simulink model "ssc_sselecpowersrc"  (R2015a)
settings: Solver=ode15s  StartTime=0.0  StopTime=3600  RelTol=1e-3
InitFcn:
  | if ~exist('E_NOM_KWH', 'var')
  |     E_NOM_KWH = 20;
  |     V_NOM = 400;
  |     E_INIT_KWH = 0.1*E_NOM_KWH;
  | end
  | 
  | C = E_NOM_KWH*3.6e6/V_NOM^2;
  | V0 = V_NOM * sqrt(2*E_INIT_KWH/E_NOM_KWH)
StopFcn:
  | clear C V0
libraries: fl_lib x7, nesl_utility x5, sselecpowersrclib x1
settings Model: Creator=e102261  LastModifiedBy=e102261
settings DataIOCC: SaveOutput=off  SignalLogging=off  DSMLogging=off  VisualizeSimOutput=off  SaveTime=off

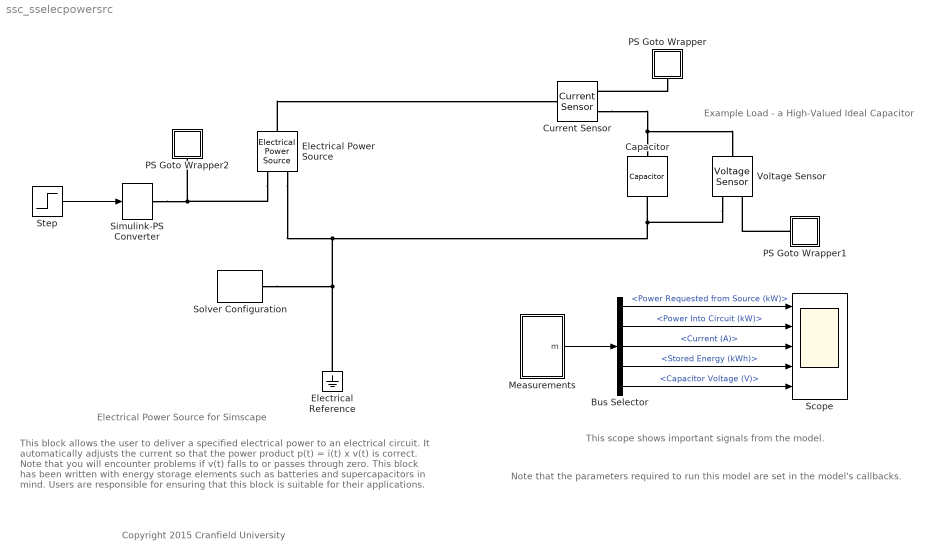
== system ssc_sselecpowersrc ==
  note: Note that the parameters required to run this model are set in the model's callbacks.
  note: This scope shows important signals from the model.
  note: Example Load - a High-Valued Ideal Capacitor
  note: This block allows the user to deliver a specified electrical power to an electrical
      | circuit. It automatically adjusts the current so that the power product
      | p(t) = i(t) x v(t) is correct.  Note that you will encounter problems if v(t) falls to or
      | passes through zero. This block has been written with energy storage elements
      | such as batteries and supercapacitors in mind. Users are responsible for
      | ensuring that this block is suitable for their applications.
  note: Copyright 2015 Cranfield University
  note: Electrical Power Source for Simscape
  Bus Selector : BusSelector  OutputSignals=Power Requested from Source (kW),Power Into Circuit (kW),Current (A),Stored Energy (kWh),Capacitor Voltage (V)
  Capacitor : fl_lib/Electrical/Electrical Elements/Capacitor  c=C F  r=0 Ohm  g=0 1/Ohm  i_specify=off  i_priority=High  i=0 A  v_specify=on  v_priority=High  v=V0 V  vc_specify=off  vc_priority=High  vc=0 V
  Current Sensor : fl_lib/Electrical/Electrical Sensors/Current Sensor
  Electrical Power Source : sselecpowersrclib/Electrical Power Source
  Electrical Reference : fl_lib/Electrical/Electrical Elements/Electrical Reference
  Measurements : Subsystem
  PS Goto Wrapper : Subsystem
  PS Goto Wrapper1 : Subsystem
  PS Goto Wrapper2 : Subsystem
  Scope : Scope  NumInputPorts=5
      settings: TimeRange=3600  YMin=0~0~0~0~0  YMax=20~20~100~10~400
  Simulink-PS Converter : nesl_utility/Simulink-PS Converter  PhysicalDomain=network_engine_domain  SubClassName=ps_input  LeftPortType=input  RightPortType=output  PseudoPeriodic=off  Frequencies=[]  NoiseDistribution=none  NoiseParameters=[]  Unit=W  AffineConversion=off  InputFiltering=off  SimscapeFilterOrder=1  InputFilterTimeConstant=0.001  UdotUserProvided=1
  Solver Configuration : nesl_utility/Solver Configuration  PhysicalDomain=network_engine_domain  SubClassName=solver  LeftPortType=input  RightPortType=generic  Accelerate=off  Tones=[]  Harmonics=[]  SimulateNoise=off  Profile=off  UseLocalSampling=off  EnableSwitchedLinearOptims=on  FrequencyDomain=off  UseCCode=off  RelTol=0.001  AbsTol=1e-06  MinStep=1e-09  ToWorkspace=off  RevertToSquareIcSolve=off  NumHomotopyIterations=100  DoDC=off  ResidualTolerance=1e-09  UseLocalSolver=off  LocalSolverChoice=NE_BACKWARD_EULER_ADVANCER  LocalSolverSampleTime=0.001  DoFixedCost=off  MaxNonlinIter=3  MaxModeIter=2  LinearAlgebra=Sparse  DelaysMemoryBudget=1024  AutomaticFiltering=on  FilteringTimeConstant=0.001
  Step : Step  Time=720  After=E_NOM_KWH/2*1e3  SampleTime=0
  Voltage Sensor : fl_lib/Electrical/Electrical Sensors/Voltage Sensor
  wires:
  Step/1 -> Simulink-PS Converter/1
  Measurements/1(m) -> Bus Selector/1
  Bus Selector/2 -> Scope/2  "<Power Into Circuit (kW)>"
  Bus Selector/1 -> Scope/1  "<Power Requested from Source (kW)>"
  Bus Selector/4 -> Scope/4  "<Stored Energy (kWh)>"
  Bus Selector/3 -> Scope/3  "<Current (A)>"
  Bus Selector/5 -> Scope/5  "<Capacitor Voltage (V)>"
  connections:
  Voltage Sensor/RConn2 -- Electrical Power Source/LConn2 -- Electrical Reference/LConn1 -- Solver Configuration/RConn1 -- Capacitor/RConn1
  Current Sensor/RConn2 -- Voltage Sensor/LConn1 -- Capacitor/LConn1
  PS Goto Wrapper1/LConn1 -- Voltage Sensor/RConn1
  Electrical Power Source/RConn1 -- Current Sensor/LConn1
  Simulink-PS Converter/RConn1 -- Electrical Power Source/LConn1 -- PS Goto Wrapper2/LConn1
  PS Goto Wrapper/LConn1 -- Current Sensor/RConn1

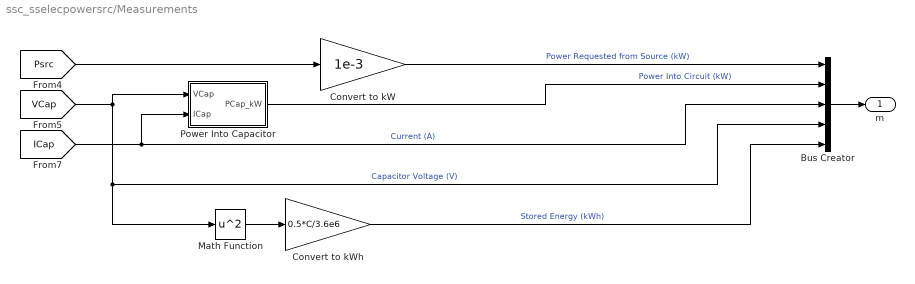
== system ssc_sselecpowersrc/Measurements ==
  Bus Creator : BusCreator  Inputs=5
  Convert to kW : Gain  Gain=1e-3
  Convert to kWh : Gain  Gain=0.5*C/3.6e6
  Math Function : Math  Operator=square  SaturateOnIntegerOverflow=on
  Power Into Capacitor : Subsystem
  m : Outport
  wires:
  Math Function/1 -> Convert to kWh/1
  Power Into Capacitor/1(PCap_kW) -> Bus Creator/2  "Power Into Circuit (kW)"
  Convert to kWh/1 -> Bus Creator/5  "Stored Energy (kWh)"
  [VCap] -> Bus Creator/4, Math Function/1, Power Into Capacitor/1(VCap)  "Capacitor Voltage (V)"
  [ICap] -> Bus Creator/3, Power Into Capacitor/2(ICap)  "Current (A)"
  [Psrc] -> Convert to kW/1
  Bus Creator/1 -> m/1
  Convert to kW/1 -> Bus Creator/1  "Power Requested from Source (kW)"

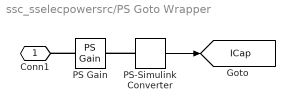
== system ssc_sselecpowersrc/PS Goto Wrapper ==
  PS Gain : fl_lib/Physical Signals/Functions/PS Gain  gain=1
  PS-Simulink Converter : nesl_utility/PS-Simulink Converter  PhysicalDomain=network_engine_domain  SubClassName=ps_output  LeftPortType=input  RightPortType=output  PseudoPeriodic=off  Frequencies=[]  Unit=A  AffineConversion=off
  Conn1 : PMIOPort  Port=1  Side=Left
  tag scope: ICap=global
  wires:
  PS-Simulink Converter/1 -> [ICap]
  connections:
  PS Gain/LConn1 -- Conn1/RConn1
  PS-Simulink Converter/LConn1 -- PS Gain/RConn1

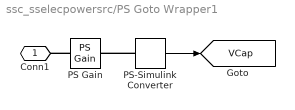
== system ssc_sselecpowersrc/PS Goto Wrapper1 ==
  PS Gain : fl_lib/Physical Signals/Functions/PS Gain  gain=1
  PS-Simulink Converter : nesl_utility/PS-Simulink Converter  PhysicalDomain=network_engine_domain  SubClassName=ps_output  LeftPortType=input  RightPortType=output  PseudoPeriodic=off  Frequencies=[]  Unit=V  AffineConversion=off
  Conn1 : PMIOPort  Port=1  Side=Left
  tag scope: VCap=global
  wires:
  PS-Simulink Converter/1 -> [VCap]
  connections:
  PS-Simulink Converter/LConn1 -- PS Gain/RConn1
  PS Gain/LConn1 -- Conn1/RConn1

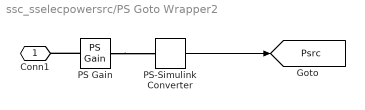
== system ssc_sselecpowersrc/PS Goto Wrapper2 ==
  PS Gain : fl_lib/Physical Signals/Functions/PS Gain  gain=1
  PS-Simulink Converter : nesl_utility/PS-Simulink Converter  PhysicalDomain=network_engine_domain  SubClassName=ps_output  LeftPortType=input  RightPortType=output  PseudoPeriodic=off  Frequencies=[]  Unit=W  AffineConversion=off
  Conn1 : PMIOPort  Port=1  Side=Left
  tag scope: Psrc=global
  wires:
  PS-Simulink Converter/1 -> [Psrc]
  connections:
  PS Gain/LConn1 -- Conn1/RConn1
  PS Gain/RConn1 -- PS-Simulink Converter/LConn1

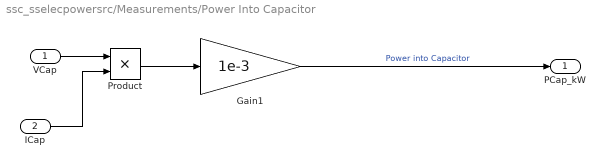
== system ssc_sselecpowersrc/Measurements/Power Into Capacitor ==
  VCap : Inport
  ICap : Inport  Port=2
  Gain1 : Gain  Gain=1e-3
  Product : Product
  PCap_kW : Outport
  wires:
  ICap/1 -> Product/2
  VCap/1 -> Product/1
  Product/1 -> Gain1/1
  Gain1/1 -> PCap_kW/1  "Power into Capacitor"
